simulink model "SF051A_SnsrOffsLrng"  (R2013b)
settings: Solver=FixedStepDiscrete  SolverMode=SingleTasking  StartTime=0.0  StopTime=1  FixedStep=0.002  RelTol=1e-3
undefined symbols (not defined in the file): ARCHGLBPRM_10MILLISEC_SEC_F32, ARCHGLBPRM_2MILLISEC_SEC_F32, ARCHGLBPRM_2PI_ULS_F32, ARCHGLBPRM_FLOATZEROTHD_ULS_F32, ARCHGLBPRM_PIOVER180_ULS_F32, CNV100MICROSECTOMILLISEC_MILLISECPERCNT_F32, CNV100MICROSECTOSEC_SECPERCNT_F32, COVRAMTRXNIT_ULS_F32, HWAUTHYTHD_ULS_F32, HWTQLRNGSTSLRND_CNT_U08, HWTQLRNGSTSNEGOFFS_CNT_U08, HWTQLRNGSTSNOTLRND_CNT_U08, HWTQLRNGSTSPOSOFFS_CNT_U08, HWTQLRNGSTSZEROOFFS_CNT_U08, HWTQLRNGTMRHILIM_SEC_F32, IDYMTRX_ULS_F32, IVS10MS_ULSPERSEC_F32, LRNGFILTICON_ULS_F32, NvmGetErrSts1, ONE_ULS_F32, SnsrOffsLrnd, SnsrOffsLrngFctEna, SnsrOffsLrngHwAgLrngDrvgDstThd, SnsrOffsLrngHwAgLrngEna, SnsrOffsLrngHwAgLrngHwVelThd, SnsrOffsLrngHwAgLrngSysTqThd, SnsrOffsLrngHwAgLrngSysTqThdMed, SnsrOffsLrngHwAgLrngSysTqThdTrustd, SnsrOffsLrngHwAgLrngSysTqThdWide, SnsrOffsLrngHwAgLrngTi, SnsrOffsLrngHwAgLrngVehSpdThd, SnsrOffsLrngHwAgLrngYawOffsDbnd, SnsrOffsLrngHwAgLrngYawRateThd, SnsrOffsLrngHwAgOffsLim, SnsrOffsLrngHwTqLrngEna, SnsrOffsLrngHwTqLrngEnaTiThd, SnsrOffsLrngHwTqLrngHwAgDbnd, SnsrOffsLrngHwTqLrngHwAgThd, SnsrOffsLrngHwTqLrngHwTqThd, SnsrOffsLrngHwTqLrngHwTqZeroOffsThd, SnsrOffsLrngHwTqLrngHwVelThd, SnsrOffsLrngHwTqLrngMeasTi, SnsrOffsLrngHwTqLrngMeasTiScar, SnsrOffsLrngHwTqLrngSampleImbThd1, SnsrOffsLrngHwTqLrngSampleImbThd2, SnsrOffsLrngHwTqLrngSampleThd1, SnsrOffsLrngHwTqLrngSampleThd2, SnsrOffsLrngHwTqLrngTiWghtCoeff, SnsrOffsLrngHwTqLrngVehSpdThd, SnsrOffsLrngHwTqOffsLim, SnsrOffsLrngSampleCntForHwTqLrngRst, SnsrOffsLrngTqInpDetnPwrEstimnThd, SnsrOffsLrngTqInpDetnSinGenrAmp, SnsrOffsLrngTqInpDetnSinGenrFrq, SnsrOffsLrngTqInpDetnStg1FilGain, SnsrOffsLrngTqInpDetnStg1WinSize, SnsrOffsLrngTqInpDetnStg2FilGainCen, SnsrOffsLrngTqInpDetnStg2FilGainDwn, SnsrOffsLrngTqInpDetnStg2FilGainUp, SnsrOffsLrngTqInpDetnStg2WinSize ... (+15)
libraries: Fil x34, FixdToFloat x17, FloatToFixd x16, NxtrLim x15, simulink x12, NxtrAbslt x12, NxtrNvM x8, NxtrMin x5, NxtrMath x3
(part 3 of 11)

== system SF051A_SnsrOffsLrng/SnsrOffsLrng/SetHwAgOffs ==
  note: User wants to force the learned offset to a particular value.  Learning will continue and then
      | be written to NVM at key off as usual.
  HwAgOffs_ArgIn : Inport
  HwAgLrngStRst_ArgIn : Inport  Port=2
  function : TriggerPort  TriggerType=function-call
  Constant1 : Constant  RequirementInfo={'linktype_rmi_doors' '0000babd (/E-STEER Core/SubSystem Specifications/Application Functions/SF051A Sensor Offset Learning)' '#SF051A_230' 'true' 'REQ:SF051A_230' '' } %GIDa_cf4a6147_0323_42ae_80d2_af4f1777b13a  Value=SnsrOffsLrngHwAgOffsLim  OutDataTypeStr=single
  Constant5 : Constant  Value=true  OutDataTypeStr=boolean
      settings: AttributesFormatString=%<OutDataTypeStr>
  Data Store Write : DataStoreWrite  DataStoreName=SnsrOffsLrnd  DataStoreElements=SnsrOffsLrnd.HwAgOffs
  Data Store Write1 : DataStoreWrite  DataStoreName=HwAgLrngStRst
  Do nothing : Subsystem  TreatAsAtomicUnit=on
  FloatToFixd_s16_f32 : FloatToFixd/FloatToFixd_s16_f32  Param1=10
  If : If  IfExpression=u1
  LimDyn_f32 : NxtrLim/LimDyn_f32  RequirementInfo={'linktype_rmi_doors' '0000babd (/E-STEER Core/SubSystem Specifications/Application Functions/SF051A Sensor Offset Learning)' '#SF051A_230' 'true' 'REQ:SF051A_230' '' } %GIDa_5bdd1159_6844_4d61_b5ac_4bd6393bb1d8
  Reset Learning : Subsystem  TreatAsAtomicUnit=on
  Set Ram Block Status : NxtrNvM/Set Ram Block Status  FuncName=Set Ram Block Status  NvMBlockName=SnsrOffsLrnd  VoidFuncRtn=on  BlockChanged_DSN=NvMSRBS_BlockChanged4  Return_DSN=NvMSRBS_Return4
      settings: AttributesFormatString=%<FuncName>
  Subsystem5 : Subsystem  Description=|  mask(Copyright Information){none=on}
      | Copyright info block.                                               
      |                                                                     
      | Place copyright information at the top of every subsystem in design.
      mask prompts: none "No parameters"
      mask help: Place copyright information at the top of every subsystem in design.
      mask Display:
      | NxtrConf = 'Nexteer Confidential';
      | 
      | sys = bdroot; %handle for the current model ("system")
      | first = get_param(sys,'Created');
      | first = first(end-3:end);  %year is last four digits
      | 
      | last = get_param(sys,'LastModifiedDate');
      | if isempty(last)
      |     last = datestr(now,'yyyy');
      | else
      |     last = last(end-3:end);
      | end
      | 
      | if strcmp(first,last)
      |     fprintf('%s -- Copyright %s Nexteer',NxtrConf,first)
      | else
      |     fprintf('%s -- %s%s- %s Nexteer',NxtrConf,char(169),first,last)
      | end
  Unary Minus : UnaryMinus  RequirementInfo={'linktype_rmi_doors' '0000babd (/E-STEER Core/SubSystem Specifications/Application Functions/SF051A Sensor Offset Learning)' '#SF051A_230' 'true' 'REQ:SF051A_230' '' } %GIDa_8391f97f_4728_4542_8e93_eb1d16ca3e52
  wires:
  Constant1/1 -> LimDyn_f32/3, Unary Minus/1
  LimDyn_f32/1 -> [SetHwAgLrngFil1StVari], FloatToFixd_s16_f32/1
  FloatToFixd_s16_f32/1 -> Data Store Write/1
  Constant5/1 -> Set Ram Block Status/1
  Unary Minus/1 -> LimDyn_f32/2
  HwAgOffs_ArgIn/1 -> LimDyn_f32/1
  [SetHwAgLrngFil1StVari] -> Reset Learning/1(SetHwAgLrngFil1StVari)
  If/1 -> Reset Learning/Action
  If/2 -> Do nothing/Action
  HwAgLrngStRst_ArgIn/1 -> Data Store Write1/1, If/1

== system SF051A_SnsrOffsLrng/SnsrOffsLrng/SetHwTqOffs ==
  note: Note for Developer:
      | This version does not have the capability of recovering
      | the last learning state once a "Reset Learning" has been
      | performed.
      | In other words: the Covariance Matriy, the Estimations Vector
      | and the Positive and Negative Counters can no be written
      | using eTool.
  note: User wants to force the learned offset to a particular value.  Learning will continue and then
      | be written to NVM at key off as usual.
  HwTqOffs_ArgIn : Inport
  HwTqLrngStRst_ArgIn : Inport  Port=2
  function : TriggerPort  TriggerType=function-call
  Constant1 : Constant  RequirementInfo={'linktype_rmi_doors' '0000babd (/E-STEER Core/SubSystem Specifications/Application Functions/SF051A Sensor Offset Learning)' '#SF051A_232' 'true' 'REQ:SF051A_232' '' } %GIDa_219fb91a_9c6b_4266_a0e9_012c6c46364f  Value=SnsrOffsLrngHwTqOffsLim  OutDataTypeStr=single
  Constant5 : Constant  Value=true  OutDataTypeStr=boolean
      settings: AttributesFormatString=%<OutDataTypeStr>
  Data Store Write : DataStoreWrite  DataStoreName=SnsrOffsLrnd  DataStoreElements=SnsrOffsLrnd.HwTqOffs
  Data Store Write1 : DataStoreWrite  DataStoreName=HwTqLrngStRst
  Do nothing : Subsystem  TreatAsAtomicUnit=on
  FloatToFixd_s16_f32 : FloatToFixd/FloatToFixd_s16_f32  Param1=12
  If : If  IfExpression=u1
  LimDyn_f32 : NxtrLim/LimDyn_f32  RequirementInfo={'linktype_rmi_doors' '0000babd (/E-STEER Core/SubSystem Specifications/Application Functions/SF051A Sensor Offset Learning)' '#SF051A_232' 'true' 'REQ:SF051A_232' '' } %GIDa_8a55e285_f6d0_4af0_87c3_e1d2354db2fa
  Reset Learning : Subsystem  TreatAsAtomicUnit=on
  Set Ram Block Status : NxtrNvM/Set Ram Block Status  FuncName=Set Ram Block Status  NvMBlockName=SnsrOffsLrnd  VoidFuncRtn=on  BlockChanged_DSN=NvMSRBS_BlockChanged5  Return_DSN=NvMSRBS_Return5
      settings: AttributesFormatString=%<FuncName>
  Subsystem5 : Subsystem  Description=|  mask(Copyright Information){none=on}
      | Copyright info block.                                               
      |                                                                     
      | Place copyright information at the top of every subsystem in design.
      mask prompts: none "No parameters"
      mask help: Place copyright information at the top of every subsystem in design.
      mask Display:
      | NxtrConf = 'Nexteer Confidential';
      | 
      | sys = bdroot; %handle for the current model ("system")
      | first = get_param(sys,'Created');
      | first = first(end-3:end);  %year is last four digits
      | 
      | last = get_param(sys,'LastModifiedDate');
      | if isempty(last)
      |     last = datestr(now,'yyyy');
      | else
      |     last = last(end-3:end);
      | end
      | 
      | if strcmp(first,last)
      |     fprintf('%s -- Copyright %s Nexteer',NxtrConf,first)
      | else
      |     fprintf('%s -- %s%s- %s Nexteer',NxtrConf,char(169),first,last)
      | end
  Unary Minus : UnaryMinus  RequirementInfo={'linktype_rmi_doors' '0000babd (/E-STEER Core/SubSystem Specifications/Application Functions/SF051A Sensor Offset Learning)' '#SF051A_232' 'true' 'REQ:SF051A_232' '' } %GIDa_49082dc0_10d2_4695_96b7_275db381282e
  wires:
  Constant1/1 -> LimDyn_f32/3, Unary Minus/1
  FloatToFixd_s16_f32/1 -> Data Store Write/1
  Constant5/1 -> Set Ram Block Status/1
  Unary Minus/1 -> LimDyn_f32/2
  HwTqOffs_ArgIn/1 -> LimDyn_f32/1
  LimDyn_f32/1 -> FloatToFixd_s16_f32/1
  If/1 -> Reset Learning/Action
  If/2 -> Do nothing/Action
  HwTqLrngStRst_ArgIn/1 -> Data Store Write1/1, If/1

== system SF051A_SnsrOffsLrng/SnsrOffsLrng/SetYawRateOffs ==
  note: User wants to force the learned offset to a particular value.  Learning will continue and then
      | be written to NVM at key off as usual.
  VehYawRateOffs_ArgIn : Inport
  VehYawRateLrngStRst_ArgIn : Inport  Port=2
  function : TriggerPort  TriggerType=function-call
  Constant1 : Constant  RequirementInfo={'linktype_rmi_doors' '0000babd (/E-STEER Core/SubSystem Specifications/Application Functions/SF051A Sensor Offset Learning)' '#SF051A_218' 'true' 'REQ:SF051A_218' '' } %GIDa_ab3e8f4a_b511_4467_8e73_7163cbff4053  Value=SnsrOffsLrngYawRateOffsLim  OutDataTypeStr=single
  Constant5 : Constant  Value=true  OutDataTypeStr=boolean
      settings: AttributesFormatString=%<OutDataTypeStr>
  Data Store Write1 : DataStoreWrite  DataStoreName=VehYawRateLrngStRst
  Do nothing : Subsystem  TreatAsAtomicUnit=on
  FloatToFixd_s16_f32 : FloatToFixd/FloatToFixd_s16_f32  Param1=9
  If : If  IfExpression=u1
  LimDyn_f32 : NxtrLim/LimDyn_f32  RequirementInfo={'linktype_rmi_doors' '0000babd (/E-STEER Core/SubSystem Specifications/Application Functions/SF051A Sensor Offset Learning)' '#SF051A_218' 'true' 'REQ:SF051A_218' '' } %GIDa_7eb17ecc_7acb_4d1e_ab0e_493e23ce8555
  NVM RAM : DataStoreWrite  DataStoreName=SnsrOffsLrnd  DataStoreElements=SnsrOffsLrnd.YawRateOffs
  Reset Learning : Subsystem  TreatAsAtomicUnit=on
  Set Ram Block Status : NxtrNvM/Set Ram Block Status  FuncName=Set Ram Block Status  NvMBlockName=SnsrOffsLrnd  VoidFuncRtn=on  BlockChanged_DSN=NvMSRBS_BlockChanged3  Return_DSN=NvMSRBS_Return3
      settings: AttributesFormatString=%<FuncName>
  Subsystem5 : Subsystem  Description=|  mask(Copyright Information){none=on}
      | Copyright info block.                                               
      |                                                                     
      | Place copyright information at the top of every subsystem in design.
      mask prompts: none "No parameters"
      mask help: Place copyright information at the top of every subsystem in design.
      mask Display:
      | NxtrConf = 'Nexteer Confidential';
      | 
      | sys = bdroot; %handle for the current model ("system")
      | first = get_param(sys,'Created');
      | first = first(end-3:end);  %year is last four digits
      | 
      | last = get_param(sys,'LastModifiedDate');
      | if isempty(last)
      |     last = datestr(now,'yyyy');
      | else
      |     last = last(end-3:end);
      | end
      | 
      | if strcmp(first,last)
      |     fprintf('%s -- Copyright %s Nexteer',NxtrConf,first)
      | else
      |     fprintf('%s -- %s%s- %s Nexteer',NxtrConf,char(169),first,last)
      | end
  Unary Minus : UnaryMinus  RequirementInfo={'linktype_rmi_doors' '0000babd (/E-STEER Core/SubSystem Specifications/Application Functions/SF051A Sensor Offset Learning)' '#SF051A_218' 'true' 'REQ:SF051A_218' '' } %GIDa_9f76f36b_b8a7_4ab3_b85e_9e0995778375
  wires:
  Constant1/1 -> Unary Minus/1, LimDyn_f32/3
  LimDyn_f32/1 -> [SetYawLrngFil1StVari], FloatToFixd_s16_f32/1
  FloatToFixd_s16_f32/1 -> NVM RAM/1
  Constant5/1 -> Set Ram Block Status/1
  Unary Minus/1 -> LimDyn_f32/2
  VehYawRateOffs_ArgIn/1 -> LimDyn_f32/1
  [SetYawLrngFil1StVari] -> Reset Learning/1(SetYawLrngFil1StVari)
  If/1 -> Reset Learning/Action
  If/2 -> Do nothing/Action
  VehYawRateLrngStRst_ArgIn/1 -> Data Store Write1/1, If/1

== system SF051A_SnsrOffsLrng/SnsrOffsLrng/SnsrOffsLrngInit1 ==
  note: Perform KUpdate operations to convert
      | calibrations from Hz to Uls
  note: If NVM is good use it as output.  Otherwise,
      | set stuff to zeros.
  function : TriggerPort  TriggerType=function-call
  Data Store Read : DataStoreRead  DataStoreName=SnsrOffsLrnd  DataStoreElements=SnsrOffsLrnd.HwTqLrngCovariMtrx(:,:)
  Display : Display
  Initialize Filters : Subsystem
  NVM Management : Subsystem
  Subsystem5 : Subsystem  Description=|  mask(Copyright Information){none=on}
      | Copyright info block.                                               
      |                                                                     
      | Place copyright information at the top of every subsystem in design.
      mask prompts: none "No parameters"
      mask help: Place copyright information at the top of every subsystem in design.
      mask Display:
      | NxtrConf = 'Nexteer Confidential';
      | 
      | sys = bdroot; %handle for the current model ("system")
      | first = get_param(sys,'Created');
      | first = first(end-3:end);  %year is last four digits
      | 
      | last = get_param(sys,'LastModifiedDate');
      | if isempty(last)
      |     last = datestr(now,'yyyy');
      | else
      |     last = last(end-3:end);
      | end
      | 
      | if strcmp(first,last)
      |     fprintf('%s -- Copyright %s Nexteer',NxtrConf,first)
      | else
      |     fprintf('%s -- %s%s- %s Nexteer',NxtrConf,char(169),first,last)
      | end
  VehYawRateOffs : Outport
  HwAgOffs : Outport  Port=2
  HwTqOffs : Outport  Port=3
  wires:
  NVM Management/1(VehYawRateOffs) -> VehYawRateOffs/1
  NVM Management/2(HwAgOffs) -> HwAgOffs/1
  NVM Management/3(HwTqOffs) -> HwTqOffs/1
  Data Store Read/1 -> Display/1

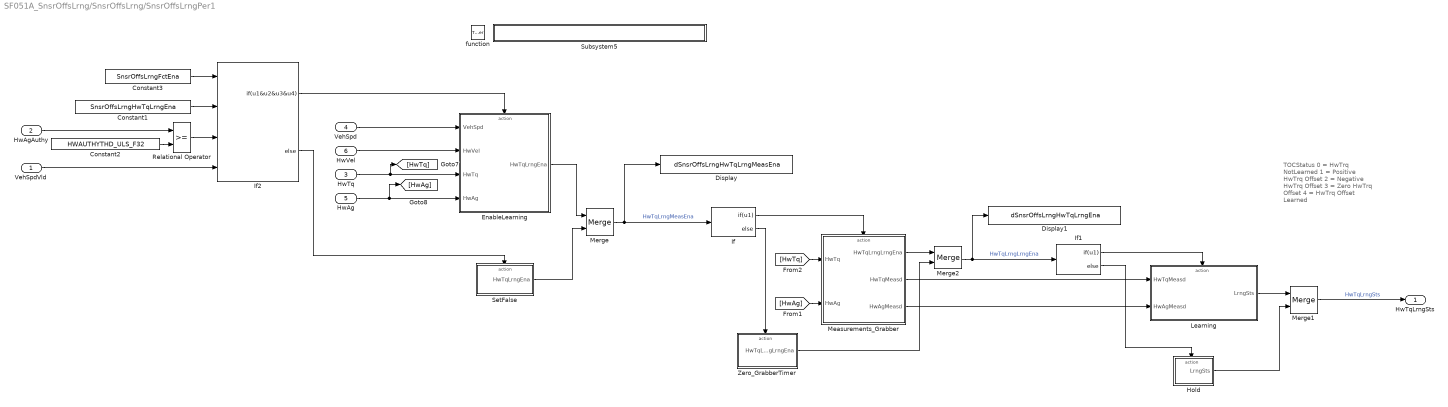
== system SF051A_SnsrOffsLrng/SnsrOffsLrng/SnsrOffsLrngPer1 ==
  note: TOCStatus
      | 0 = HwTrq NotLearned
      | 1 = Positive HwTrq Offset
      | 2 = Negative HwTrq Offset
      | 3 = Zero HwTrq Offset
      | 4 = HwTrq Offset Learned
  VehSpdVld : Inport  RequirementInfo={'linktype_rmi_doors' '0000babd (/E-STEER Core/SubSystem Specifications/Application Functions/SF051A Sensor Offset Learning)' '#SF051A_172' 'true' 'REQ:SF051A_172' '' } %GIDa_4c8f98fb_59b3_4f0f_a449_e0f476a92c6b
  HwAgAuthy : Inport  RequirementInfo={'linktype_rmi_doors' '0000babd (/E-STEER Core/SubSystem Specifications/Application Functions/SF051A Sensor Offset Learning)' '#SF051A_172' 'true' 'REQ:SF051A_172' '' } %GIDa_bc799a18_930e_49aa_970e_d738f90c29be  Port=2
  HwTq : Inport  RequirementInfo={'linktype_rmi_doors' '0000babd (/E-STEER Core/SubSystem Specifications/Application Functions/SF051A Sensor Offset Learning)' '#SF051A_168' 'true' 'REQ:SF051A_168' '' } %GIDa_0cdb420e_6740_4194_bc6e_307440cdb44a  Port=3
  VehSpd : Inport  RequirementInfo={'linktype_rmi_doors' '0000babd (/E-STEER Core/SubSystem Specifications/Application Functions/SF051A Sensor Offset Learning)' '#SF051A_171' 'true' 'REQ:SF051A_171' '' } %GIDa_39046408_4297_4feb_8dd1_f49d24eac858  Port=4
  HwAg : Inport  RequirementInfo={'linktype_rmi_doors' '0000babd (/E-STEER Core/SubSystem Specifications/Application Functions/SF051A Sensor Offset Learning)' '#SF051A_170' 'true' 'REQ:SF051A_170' '' } %GIDa_3e08615c_a8b7_4c69_ae09_e09287af3916  Port=5
  HwVel : Inport  RequirementInfo={'linktype_rmi_doors' '0000babd (/E-STEER Core/SubSystem Specifications/Application Functions/SF051A Sensor Offset Learning)' '#SF051A_169' 'true' 'REQ:SF051A_169' '' } %GIDa_81a5698e_2e55_4c38_b0b0_32579241a4a2  Port=6
  function : TriggerPort  TriggerType=function-call
  Constant1 : Constant  RequirementInfo={'linktype_rmi_doors' '0000babd (/E-STEER Core/SubSystem Specifications/Application Functions/SF051A Sensor Offset Learning)' '#SF051A_149' 'true' 'REQ:SF051A_149' '' ; 'linktype_rmi_doors' '0000babd (/E-STEER Core/SubSystem Specifications/Application Functions/SF051A Sensor Offset Learning)' '#SF051A_172' 'true' 'REQ:SF051A_172' '' } %GIDa_535f024a_9979_46f7_87c9_cdf0e6070b24  Value=SnsrOffsLrngHwTqLrngEna
  Constant2 : Constant  RequirementInfo={'linktype_rmi_doors' '0000babd (/E-STEER Core/SubSystem Specifications/Application Functions/SF051A Sensor Offset Learning)' '#SF051A_172' 'true' 'REQ:SF051A_172' '' } %GIDa_122749e3_4a4e_4ab2_967d_239078c81b67  Value=HWAUTHYTHD_ULS_F32
  Constant3 : Constant  RequirementInfo={'linktype_rmi_doors' '0000babd (/E-STEER Core/SubSystem Specifications/Application Functions/SF051A Sensor Offset Learning)' '#SF051A_26' 'true' 'REQ:SF051A_26' '' } %GIDa_da187dda_b310_4c1b_bb0d_bc714549b8f1  Value=SnsrOffsLrngFctEna
  Display : DataStoreWrite  DataStoreName=dSnsrOffsLrngHwTqLrngMeasEna
  Display1 : DataStoreWrite  DataStoreName=dSnsrOffsLrngHwTqLrngEna
  EnableLearning : Subsystem  RequirementInfo={'linktype_rmi_doors' '0000babd (/E-STEER Core/SubSystem Specifications/Application Functions/SF051A Sensor Offset Learning)' '#SF051A_165' 'true' 'REQ:SF051A_165' '' } %GIDa_b1222e97_8db5_4cd5_9a17_e480f73facda  TreatAsAtomicUnit=on
  Hold : Subsystem  TreatAsAtomicUnit=on
  If : If  RequirementInfo={'linktype_rmi_doors' '0000babd (/E-STEER Core/SubSystem Specifications/Application Functions/SF051A Sensor Offset Learning)' '#SF051A_162' 'true' 'REQ:SF051A_162' '' } %GIDa_ff422a66_a1c6_4a1f_8e22_e07d1158d789  IfExpression=u1
  If1 : If  RequirementInfo={'linktype_rmi_doors' '0000babd (/E-STEER Core/SubSystem Specifications/Application Functions/SF051A Sensor Offset Learning)' '#SF051A_182' 'true' 'REQ:SF051A_182' '' } %GIDa_2b1810eb_40e4_47d2_bf1d_d63a9f5ada2e  IfExpression=u1
  If2 : If  RequirementInfo={'linktype_rmi_doors' '0000babd (/E-STEER Core/SubSystem Specifications/Application Functions/SF051A Sensor Offset Learning)' '#SF051A_172' 'true' 'REQ:SF051A_172' '' ; 'linktype_rmi_doors' '0000babd (/E-STEER Core/SubSystem Specifications/Application Functions/SF051A Sensor Offset Learning)' '#SF051A_26' 'true' 'REQ:SF051A_26' '' } %GIDa_c02bc2c0_3e44_40e5_864a_39991bb27631  NumInputs=4  IfExpression=u1&u2&u3&u4
  Learning : Subsystem  RequirementInfo={'linktype_rmi_doors' '0000babd (/E-STEER Core/SubSystem Specifications/Application Functions/SF051A Sensor Offset Learning)' '#SF051A_167' 'true' 'REQ:SF051A_167' '' ; 'linktype_rmi_doors' '0000babd (/E-STEER Core/SubSystem Specifications/Application Functions/SF051A Sensor Offset Learning)' '#SF051A_152' 'true' 'REQ:SF051A_152' '' } %GIDa_1b59b871_a124_470c_ac32_3b22f2dc3167  TreatAsAtomicUnit=on
  Measurements_Grabber : Subsystem  RequirementInfo={'linktype_rmi_doors' '0000babd (/E-STEER Core/SubSystem Specifications/Application Functions/SF051A Sensor Offset Learning)' '#SF051A_163' 'true' 'REQ:SF051A_163' '' } %GIDa_6482af8e_2bfa_4ab1_8618_42b9ef0606fb  TreatAsAtomicUnit=on
  Merge : Merge
  Merge1 : Merge
  Merge2 : Merge
  Relational Operator : RelationalOperator  RequirementInfo={'linktype_rmi_doors' '0000babd (/E-STEER Core/SubSystem Specifications/Application Functions/SF051A Sensor Offset Learning)' '#SF051A_172' 'true' 'REQ:SF051A_172' '' } %GIDa_037935c3_3c71_42e9_a97d_8c93dc2f08bc  OutDataTypeStr=boolean
  SetFalse : Subsystem  TreatAsAtomicUnit=on
  Subsystem5 : Subsystem  Description=|  mask(Copyright Information){none=on}
      | Copyright info block.                                               
      |                                                                     
      | Place copyright information at the top of every subsystem in design.
      mask prompts: none "No parameters"
      mask help: Place copyright information at the top of every subsystem in design.
      mask Display:
      | NxtrConf = 'Nexteer Confidential';
      | 
      | sys = bdroot; %handle for the current model ("system")
      | first = get_param(sys,'Created');
      | first = first(end-3:end);  %year is last four digits
      | 
      | last = get_param(sys,'LastModifiedDate');
      | if isempty(last)
      |     last = datestr(now,'yyyy');
      | else
      |     last = last(end-3:end);
      | end
      | 
      | if strcmp(first,last)
      |     fprintf('%s -- Copyright %s Nexteer',NxtrConf,first)
      | else
      |     fprintf('%s -- %s%s- %s Nexteer',NxtrConf,char(169),first,last)
      | end
  Zero_GrabberTimer : Subsystem  TreatAsAtomicUnit=on
  HwTqLrngSts : Outport
  wires:
  Relational Operator/1 -> If2/3
  VehSpdVld/1 -> If2/4
  HwAgAuthy/1 -> Relational Operator/1
  Constant2/1 -> Relational Operator/2
  Constant3/1 -> If2/1
  VehSpd/1 -> EnableLearning/1(VehSpd)
  HwVel/1 -> EnableLearning/2(HwVel)
  If/1 -> Measurements_Grabber/Action
  If/2 -> Zero_GrabberTimer/Action
  Measurements_Grabber/1(HwTqLrngLrngEna) -> Merge2/1
  Measurements_Grabber/2(" HwTqMeasd") -> Learning/1(HwTqMeasd)
  Measurements_Grabber/3(HwAgMeasd) -> Learning/2(HwAgMeasd)
  If1/1 -> Learning/Action
  Merge1/1 -> HwTqLrngSts/1  "HwTqLrngSts"
  Constant1/1 -> If2/2
  If2/1 -> EnableLearning/Action
  If2/2 -> SetFalse/Action
  SetFalse/1(HwTqLrngEna) -> Merge/2
  EnableLearning/1(HwTqLrngEna) -> Merge/1
  Merge/1 -> If/1, Display/1  "HwTqLrngMeasEna"
  If1/2 -> Hold/Action
  Learning/1(LrngSts) -> Merge1/1
  Hold/1(LrngSts) -> Merge1/2
  [HwAg] -> Measurements_Grabber/2(HwAg)
  [HwTq] -> Measurements_Grabber/1(HwTq)
  Merge2/1 -> Display1/1, If1/1  "HwTqLrngLrngEna"
  Zero_GrabberTimer/1(HwTqLrngLrngEna) -> Merge2/2
  HwTq/1 -> [HwTq], EnableLearning/3(HwTq)
  HwAg/1 -> [HwAg], EnableLearning/4(HwAg)

== system SF051A_SnsrOffsLrng/SnsrOffsLrng/SnsrOffsLrngPer2 ==
  VehSpd : Inport
  HwAg : Inport  Port=2
  VehYawRate : Inport  Port=3
  HwVel : Inport  Port=4
  HwTq : Inport  Port=5
  MotTqCmdCrf : Inport  Port=6
  VehYawRateVld : Inport  Port=7
  HwAgAuthy : Inport  Port=8
  VehSpedVld : Inport  Port=9
  HwTqLrngSts : Inport  Port=10
  function : TriggerPort  TriggerType=function-call
  Constant : Constant  RequirementInfo={'linktype_rmi_doors' '0000babd (/E-STEER Core/SubSystem Specifications/Application Functions/SF051A Sensor Offset Learning)' '#SF051A_26' 'true' 'REQ:SF051A_26' '' } %GIDa_87a2c3d1_22c0_4f41_9628_e13acbd87715  Value=SnsrOffsLrngFctEna
  Do nothing : Subsystem  TreatAsAtomicUnit=on
  Enable_Function : Subsystem  TreatAsAtomicUnit=on
  If : If  RequirementInfo={'linktype_rmi_doors' '0000babd (/E-STEER Core/SubSystem Specifications/Application Functions/SF051A Sensor Offset Learning)' '#SF051A_26' 'true' 'REQ:SF051A_26' '' } %GIDa_ccb961ec_3e2e_4777_9fe3_5289931ee51d  IfExpression=u1
  Subsystem5 : Subsystem  Description=|  mask(Copyright Information){none=on}
      | Copyright info block.                                               
      |                                                                     
      | Place copyright information at the top of every subsystem in design.
      mask prompts: none "No parameters"
      mask help: Place copyright information at the top of every subsystem in design.
      mask Display:
      | NxtrConf = 'Nexteer Confidential';
      | 
      | sys = bdroot; %handle for the current model ("system")
      | first = get_param(sys,'Created');
      | first = first(end-3:end);  %year is last four digits
      | 
      | last = get_param(sys,'LastModifiedDate');
      | if isempty(last)
      |     last = datestr(now,'yyyy');
      | else
      |     last = last(end-3:end);
      | end
      | 
      | if strcmp(first,last)
      |     fprintf('%s -- Copyright %s Nexteer',NxtrConf,first)
      | else
      |     fprintf('%s -- %s%s- %s Nexteer',NxtrConf,char(169),first,last)
      | end
  wires:
  VehSpd/1 -> Enable_Function/1(VehSpd)
  HwAg/1 -> Enable_Function/2(HwAg)
  VehYawRate/1 -> Enable_Function/3(VehYawRate)
  HwVel/1 -> Enable_Function/4(HwVel)
  HwTq/1 -> Enable_Function/5(HwTq)
  MotTqCmdCrf/1 -> Enable_Function/6(MotTqCmdCrf)
  VehYawRateVld/1 -> Enable_Function/7(VehYawRateVld)
  HwAgAuthy/1 -> Enable_Function/8(HwAgAuthy)
  VehSpedVld/1 -> Enable_Function/9(VehSpedVld)
  HwTqLrngSts/1 -> Enable_Function/10(HwTqLrngSts)
  Constant/1 -> If/1
  If/1 -> Enable_Function/Action
  If/2 -> Do nothing/Action

== system SF051A_SnsrOffsLrng/SnsrOffsLrng/Subsystem5 ==

== system SF051A_SnsrOffsLrng/call_SnsrOffsLrngInit1/Subsystem5 ==

== system SF051A_SnsrOffsLrng/call_SnsrOffsLrngPer1/Subsystem5 ==

== system SF051A_SnsrOffsLrng/call_SnsrOffsLrngPer2/Subsystem5 ==

== system SF051A_SnsrOffsLrng/SnsrOffsLrng/GetHwAgOffs/Subsystem5 ==

== system SF051A_SnsrOffsLrng/SnsrOffsLrng/GetHwTqOffs/Subsystem5 ==

== system SF051A_SnsrOffsLrng/SnsrOffsLrng/GetYawRateOffs/Subsystem5 ==

== system SF051A_SnsrOffsLrng/SnsrOffsLrng/RstHwTq/GetRefTmr100MicroSec32bit ==
  note: 1 count = 100 uSec
  note: seconds
  note: microseconds
  note: counts
  note: Wrap-to-zero
  note: GetRefTmr100MicroSec32bit
  note: Created Aug 18, 2015
      | Modified Oct 21, 2015
      | Modified Oct 30, 2015
      | Kevin Derry
  CopyRight2 : Subsystem  Description=|  mask(Copyright Information){none=on}
      | Copyright info block.                                               
      |                                                                     
      | Place copyright information at the top of every subsystem in design.
      mask prompts: none "No parameters"
      mask help: Place copyright information at the top of every subsystem in design.
      mask Display:
      | NxtrConf = 'Nexteer Confidential';
      | 
      | sys = bdroot; %handle for the current model ("system")
      | first = get_param(sys,'Created');
      | if(isempty(first))
      |     first = datestr(now,'yyyy');
      | else
      |     first = first(end-3:end);  %year is last four digits
      | end
      | 
      | last = get_param(sys,'LastModifiedDate');
      | if isempty(last)
      |     last = datestr(now,'yyyy');
      | else
      |     last = last(end-3:end);
      | end
      | 
      | if strcmp(first,last)
      |     fprintf('%s -- Copyright %s Nexteer',NxtrConf,first)
      | else
      |     fprintf('%s -- %s%s- %s Nexteer',NxtrConf,char(169),first,last)
      | end
  Count per uSec : Constant  Value=0.01
  Data Store Read1 : DataStoreRead  DataStoreName=SimnTi
  Data Type Conversion1 : DataTypeConversion  OutDataTypeStr=uint32
  Divide1 : Product  Inputs=**
  Divide2 : Product  Inputs=*/
  Max Counts : Constant  Value=2^32-1
  Product1 : Product
  Product2 : Product
  Rounding : Rounding
  Subtract1 : Sum  Inputs=+-
  uSec per Sec : Constant  Value=1000000
  RefTmr : Outport
  wires:
  Product2/1 -> Subtract1/2
  Subtract1/1 -> Data Type Conversion1/1
  Rounding/1 -> Product2/1
  Divide2/1 -> Rounding/1
  Max Counts/1 -> Divide2/2, Product2/2
  Divide1/1 -> Divide2/1, Subtract1/1
  Product1/1 -> Divide1/1
  Count per uSec/1 -> Divide1/2
  uSec per Sec/1 -> Product1/2
  Data Type Conversion1/1 -> RefTmr/1
  Data Store Read1/1 -> Product1/1

== system SF051A_SnsrOffsLrng/SnsrOffsLrng/RstHwTq/Subsystem5 ==

== system SF051A_SnsrOffsLrng/SnsrOffsLrng/RstYawAndAg/Subsystem5 ==

== system SF051A_SnsrOffsLrng/SnsrOffsLrng/SetHwAgOffs/Do nothing ==
  Action Port : ActionPort  ActionType=else
  Subsystem5 : Subsystem  Description=|  mask(Copyright Information){none=on}
      | Copyright info block.                                               
      |                                                                     
      | Place copyright information at the top of every subsystem in design.
      mask prompts: none "No parameters"
      mask help: Place copyright information at the top of every subsystem in design.
      mask Display:
      | NxtrConf = 'Nexteer Confidential';
      | 
      | sys = bdroot; %handle for the current model ("system")
      | first = get_param(sys,'Created');
      | first = first(end-3:end);  %year is last four digits
      | 
      | last = get_param(sys,'LastModifiedDate');
      | if isempty(last)
      |     last = datestr(now,'yyyy');
      | else
      |     last = last(end-3:end);
      | end
      | 
      | if strcmp(first,last)
      |     fprintf('%s -- Copyright %s Nexteer',NxtrConf,first)
      | else
      |     fprintf('%s -- %s%s- %s Nexteer',NxtrConf,char(169),first,last)
      | end

== system SF051A_SnsrOffsLrng/SnsrOffsLrng/SetHwAgOffs/Reset Learning ==
  SetHwAgLrngFil1StVari : Inport
  Action Port : ActionPort  ActionType=then
  Constant : Constant  Value=ZERO_ULS_F32  OutDataTypeStr=single
      settings: AttributesFormatString=%<OutDataTypeStr>
  Constant1 : Constant  Value=ZERO_ULS_F32  OutDataTypeStr=single
      settings: AttributesFormatString=%<OutDataTypeStr>
  Constant2 : Constant  Value=0  OutDataTypeStr=int16
      settings: AttributesFormatString=%<OutDataTypeStr>
  Data Store Write : DataStoreWrite  DataStoreName=HwAgLrngFil1  DataStoreElements=HwAgLrngFil1.FilSt
  Data Store Write1 : DataStoreWrite  DataStoreName=HwAgLrngSysTqFil1  DataStoreElements=HwAgLrngSysTqFil1.FilSt
  Data Store Write2 : DataStoreWrite  DataStoreName=SnsrOffsLrnd  DataStoreElements=SnsrOffsLrnd.HwAgLrndTi#SnsrOffsLrnd.HwAgLrngHwAgFilSt#SnsrOffsLrnd.HwAgLrngSysTqFilSt#SnsrOffsLrnd.HwAgLrngYawOffsRef
  Data Store Write3 : DataStoreWrite  DataStoreName=HwAgLrngFil2  DataStoreElements=HwAgLrngFil2.FilSt
  Data Store Write4 : DataStoreWrite  DataStoreName=HwAgLrngSysTqFil2  DataStoreElements=HwAgLrngSysTqFil2.FilSt
  NVM Read : DataStoreRead  DataStoreName=SnsrOffsLrnd  DataStoreElements=SnsrOffsLrnd.YawRateOffs
  Subsystem5 : Subsystem  Description=|  mask(Copyright Information){none=on}
      | Copyright info block.                                               
      |                                                                     
      | Place copyright information at the top of every subsystem in design.
      mask prompts: none "No parameters"
      mask help: Place copyright information at the top of every subsystem in design.
      mask Display:
      | NxtrConf = 'Nexteer Confidential';
      | 
      | sys = bdroot; %handle for the current model ("system")
      | first = get_param(sys,'Created');
      | first = first(end-3:end);  %year is last four digits
      | 
      | last = get_param(sys,'LastModifiedDate');
      | if isempty(last)
      |     last = datestr(now,'yyyy');
      | else
      |     last = last(end-3:end);
      | end
      | 
      | if strcmp(first,last)
      |     fprintf('%s -- Copyright %s Nexteer',NxtrConf,first)
      | else
      |     fprintf('%s -- %s%s- %s Nexteer',NxtrConf,char(169),first,last)
      | end
  wires:
  SetHwAgLrngFil1StVari/1 -> Data Store Write3/1, Data Store Write/1
  Constant/1 -> Data Store Write4/1, Data Store Write1/1
  Constant1/1 -> Data Store Write2/1
  NVM Read/1 -> Data Store Write2/4
  Constant2/1 -> Data Store Write2/3, Data Store Write2/2

== system SF051A_SnsrOffsLrng/SnsrOffsLrng/SetHwAgOffs/Subsystem5 ==

== system SF051A_SnsrOffsLrng/SnsrOffsLrng/SetHwTqOffs/Do nothing ==
  Action Port : ActionPort  ActionType=else
  Subsystem5 : Subsystem  Description=|  mask(Copyright Information){none=on}
      | Copyright info block.                                               
      |                                                                     
      | Place copyright information at the top of every subsystem in design.
      mask prompts: none "No parameters"
      mask help: Place copyright information at the top of every subsystem in design.
      mask Display:
      | NxtrConf = 'Nexteer Confidential';
      | 
      | sys = bdroot; %handle for the current model ("system")
      | first = get_param(sys,'Created');
      | first = first(end-3:end);  %year is last four digits
      | 
      | last = get_param(sys,'LastModifiedDate');
      | if isempty(last)
      |     last = datestr(now,'yyyy');
      | else
      |     last = last(end-3:end);
      | end
      | 
      | if strcmp(first,last)
      |     fprintf('%s -- Copyright %s Nexteer',NxtrConf,first)
      | else
      |     fprintf('%s -- %s%s- %s Nexteer',NxtrConf,char(169),first,last)
      | end

== system SF051A_SnsrOffsLrng/SnsrOffsLrng/SetHwTqOffs/Reset Learning ==
  note: LPFs
  note: State Variables
  note: NVM
  Action Port : ActionPort  ActionType=then
  Constant1 : Constant  Value=ZERO_ULS_F32  OutDataTypeStr=single
      settings: AttributesFormatString=%<OutDataTypeStr>
  Constant10 : Constant  Value=true  OutDataTypeStr=boolean
      settings: AttributesFormatString=%<OutDataTypeStr>
  Constant3 : Constant  Value=SYSGLBPRM_HWAGHILIM_HWDEG_F32  OutDataTypeStr=single
      settings: AttributesFormatString=%<OutDataTypeStr>
  Constant4 : Constant  Value=IDYMTRX_ULS_F32  VectorParams1D=off  OutDataTypeStr=single
      settings: AttributesFormatString=%<OutDataTypeStr>, 3x3
  Constant5 : Constant  Value=0  OutDataTypeStr=uint16
      settings: AttributesFormatString=%<OutDataTypeStr>
  Constant6 : Constant  Value=0  OutDataTypeStr=uint8
      settings: AttributesFormatString=%<OutDataTypeStr>
  Constant7 : Constant  Value=ZEROVECT_ULS_F32  VectorParams1D=off  OutDataTypeStr=single
      settings: AttributesFormatString=%<OutDataTypeStr>, 3x1
  Constant8 : Constant  Value=COVRAMTRXNIT_ULS_F32  OutDataTypeStr=single
      settings: AttributesFormatString=%<OutDataTypeStr>
  Constant9 : Constant  Value=false  OutDataTypeStr=boolean
      settings: AttributesFormatString=%<OutDataTypeStr>
  Data Store Write1 : DataStoreWrite  DataStoreName=HwTqLrngEnaTmrRef
  Data Store Write10 : DataStoreWrite  DataStoreName=HwTqLrngTqInpPrsnt
  Data Store Write2 : DataStoreWrite  DataStoreName=HwTqLrngMeasTmrRef
  Data Store Write4 : DataStoreWrite  DataStoreName=HwAgMeasFil1  DataStoreElements=HwAgMeasFil1.FilSt
  Data Store Write5 : DataStoreWrite  DataStoreName=HwAgMeasFil2  DataStoreElements=HwAgMeasFil2.FilSt
  Data Store Write6 : DataStoreWrite  DataStoreName=HwTqMeasFil1  DataStoreElements=HwTqMeasFil1.FilSt
  Data Store Write7 : DataStoreWrite  DataStoreName=HwTqMeasFil2  DataStoreElements=HwTqMeasFil2.FilSt
  Data Store Write8 : DataStoreWrite  DataStoreName=HwTqLrngTqInpDetnEnaPrev
  Data Store Write9 : DataStoreWrite  DataStoreName=TqInpDetnHwTqFil  DataStoreElements=TqInpDetnHwTqFil.FilSt
  FloatToFixd_s16_f32 : FloatToFixd/FloatToFixd_s16_f32  Param1=4
  GetRefTmr100MicroSec32bit : Subsystem
  Product : Product
  Subsystem5 : Subsystem  Description=|  mask(Copyright Information){none=on}
      | Copyright info block.                                               
      |                                                                     
      | Place copyright information at the top of every subsystem in design.
      mask prompts: none "No parameters"
      mask help: Place copyright information at the top of every subsystem in design.
      mask Display:
      | NxtrConf = 'Nexteer Confidential';
      | 
      | sys = bdroot; %handle for the current model ("system")
      | first = get_param(sys,'Created');
      | first = first(end-3:end);  %year is last four digits
      | 
      | last = get_param(sys,'LastModifiedDate');
      | if isempty(last)
      |     last = datestr(now,'yyyy');
      | else
      |     last = last(end-3:end);
      | end
      | 
      | if strcmp(first,last)
      |     fprintf('%s -- Copyright %s Nexteer',NxtrConf,first)
      | else
      |     fprintf('%s -- %s%s- %s Nexteer',NxtrConf,char(169),first,last)
      | end
  Update NVM RAM : DataStoreWrite  DataStoreName=SnsrOffsLrnd  DataStoreElements=SnsrOffsLrnd.HwTqLrngSampleCntNeg#SnsrOffsLrnd.HwTqLrngSampleCntPos#SnsrOffsLrnd.HwTqLrngSts#SnsrOffsLrnd.HwTqLrngHwAgRef#SnsrOffsLrnd.HwTqLrngEstimnVect(:,:)#SnsrOffsLrnd.HwTqLrngCovariMtrx(:,:)
  wires:
  Constant1/1 -> Data Store Write9/1, Data Store Write7/1, Data Store Write6/1, Data Store Write5/1, Data Store Write4/1
  GetRefTmr100MicroSec32bit/1(RefTmr) -> Data Store Write2/1, Data Store Write1/1
  Constant3/1 -> FloatToFixd_s16_f32/1
  Constant5/1 -> Update NVM RAM/2, Update NVM RAM/1
  Constant6/1 -> Update NVM RAM/3
  Constant7/1 -> Update NVM RAM/5
  Constant4/1 -> Product/1
  Constant8/1 -> Product/2
  Product/1 -> Update NVM RAM/6
  Constant9/1 -> Data Store Write8/1
  Constant10/1 -> Data Store Write10/1
  FloatToFixd_s16_f32/1 -> Update NVM RAM/4

== system SF051A_SnsrOffsLrng/SnsrOffsLrng/SetHwTqOffs/Subsystem5 ==

== system SF051A_SnsrOffsLrng/SnsrOffsLrng/SetYawRateOffs/Do nothing ==
  Action Port : ActionPort  ActionType=else
  Subsystem5 : Subsystem  Description=|  mask(Copyright Information){none=on}
      | Copyright info block.                                               
      |                                                                     
      | Place copyright information at the top of every subsystem in design.
      mask prompts: none "No parameters"
      mask help: Place copyright information at the top of every subsystem in design.
      mask Display:
      | NxtrConf = 'Nexteer Confidential';
      | 
      | sys = bdroot; %handle for the current model ("system")
      | first = get_param(sys,'Created');
      | first = first(end-3:end);  %year is last four digits
      | 
      | last = get_param(sys,'LastModifiedDate');
      | if isempty(last)
      |     last = datestr(now,'yyyy');
      | else
      |     last = last(end-3:end);
      | end
      | 
      | if strcmp(first,last)
      |     fprintf('%s -- Copyright %s Nexteer',NxtrConf,first)
      | else
      |     fprintf('%s -- %s%s- %s Nexteer',NxtrConf,char(169),first,last)
      | end

== system SF051A_SnsrOffsLrng/SnsrOffsLrng/SetYawRateOffs/Reset Learning ==
  note: Length of time since last learned.
  note: Length of time spent learning.
  SetYawLrngFil1StVari : Inport
  Action Port : ActionPort  ActionType=then
  Constant : Constant  Value=ZERO_ULS_F32  OutDataTypeStr=single
      settings: AttributesFormatString=%<OutDataTypeStr>
  Data Store Write1 : DataStoreWrite  DataStoreName=YawLrngElpdLrngTi
  Data Store Write2 : DataStoreWrite  DataStoreName=SnsrOffsLrnd  DataStoreElements=SnsrOffsLrnd.YawRateElpdTi
  Data Store Write3 : DataStoreWrite  DataStoreName=YawLrngFil2  DataStoreElements=YawLrngFil2.FilSt
  Data Store Write4 : DataStoreWrite  DataStoreName=YawLrngFil1  DataStoreElements=YawLrngFil1.FilSt
  Subsystem5 : Subsystem  Description=|  mask(Copyright Information){none=on}
      | Copyright info block.                                               
      |                                                                     
      | Place copyright information at the top of every subsystem in design.
      mask prompts: none "No parameters"
      mask help: Place copyright information at the top of every subsystem in design.
      mask Display:
      | NxtrConf = 'Nexteer Confidential';
      | 
      | sys = bdroot; %handle for the current model ("system")
      | first = get_param(sys,'Created');
      | first = first(end-3:end);  %year is last four digits
      | 
      | last = get_param(sys,'LastModifiedDate');
      | if isempty(last)
      |     last = datestr(now,'yyyy');
      | else
      |     last = last(end-3:end);
      | end
      | 
      | if strcmp(first,last)
      |     fprintf('%s -- Copyright %s Nexteer',NxtrConf,first)
      | else
      |     fprintf('%s -- %s%s- %s Nexteer',NxtrConf,char(169),first,last)
      | end
  wires:
  SetYawLrngFil1StVari/1 -> Data Store Write3/1, Data Store Write4/1
  Constant/1 -> Data Store Write2/1, Data Store Write1/1

== system SF051A_SnsrOffsLrng/SnsrOffsLrng/SetYawRateOffs/Subsystem5 ==

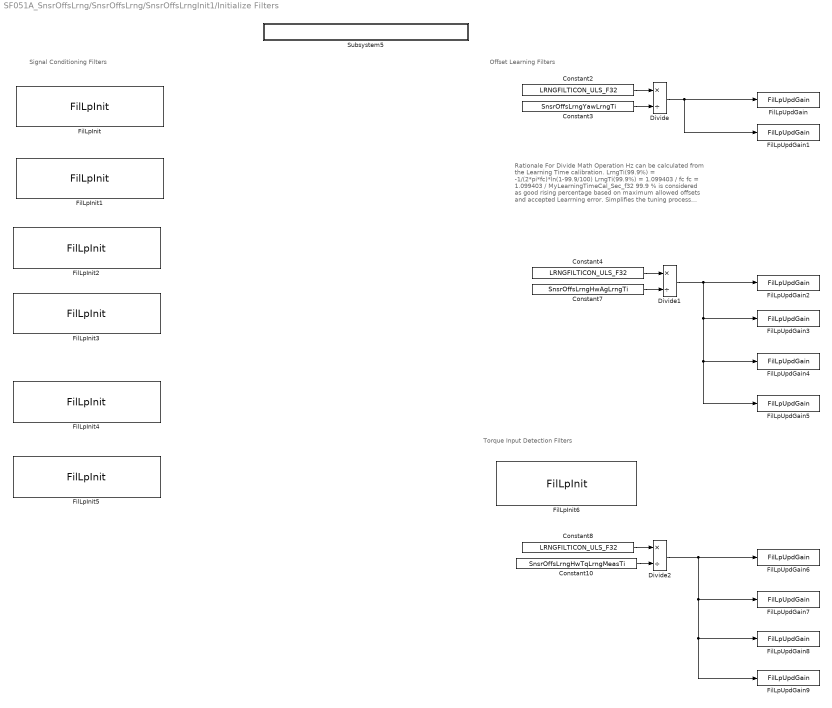
== system SF051A_SnsrOffsLrng/SnsrOffsLrng/SnsrOffsLrngInit1/Initialize Filters ==
  note: Rationale For Divide Math Operation
      |   Hz can be calculated from the Learning Time calibration.
      |   LrngTi(99.9%) = -1/(2*pi*fc)*ln(1-99.9/100)
      |   LrngTi(99.9%) = 1.099403 / fc
      |   fc = 1.099403 / MyLearningTimeCal_Sec_f32
      |
      |   99.9 % is considered as good rising percentage based on
      |   maximum allowed offsets and accepted Learrning error.
      |   Simplifies the tuning process and prevents the customer to
      |   directly find out that we use LPF as the learning method.
  note: Signal Conditioning Filters
  note: Offset Learning Filters
  note: Torque Input Detection Filters
  Constant10 : Constant  Value=SnsrOffsLrngHwTqLrngMeasTi
  Constant2 : Constant  Value=LRNGFILTICON_ULS_F32
  Constant3 : Constant  Value=SnsrOffsLrngYawLrngTi
  Constant4 : Constant  Value=LRNGFILTICON_ULS_F32
  Constant7 : Constant  Value=SnsrOffsLrngHwAgLrngTi
  Constant8 : Constant  Value=LRNGFILTICON_ULS_F32
  Divide : Product  Inputs=*/
  Divide1 : Product  Inputs=*/
  Divide2 : Product  Inputs=*/
  FilLpInit : Fil/FilLpInit  Ic=0  Ts=ARCHGLBPRM_10MILLISEC_SEC_F32  Freq=SnsrOffsLrngYawRateCdngFilFrq  StVar=YawCdngFil1
  FilLpInit1 : Fil/FilLpInit  Ic=0  Ts=ARCHGLBPRM_10MILLISEC_SEC_F32  Freq=SnsrOffsLrngYawRateCdngFilFrq  StVar=YawCdngFil2
  FilLpInit2 : Fil/FilLpInit  Ic=0  Ts=ARCHGLBPRM_10MILLISEC_SEC_F32  Freq=SnsrOffsLrngYawACdngFilFrq  StVar=YawACdngFil
  FilLpInit3 : Fil/FilLpInit  Ic=0  Ts=ARCHGLBPRM_10MILLISEC_SEC_F32  Freq=SnsrOffsLrngTqAndAgFilFrq  StVar=HwAgCdngFil
  FilLpInit4 : Fil/FilLpInit  Ic=0  Ts=ARCHGLBPRM_10MILLISEC_SEC_F32  Freq=SnsrOffsLrngHwVelFilFrq  StVar=HwVelCdngFil
  FilLpInit5 : Fil/FilLpInit  Ic=0  Ts=ARCHGLBPRM_10MILLISEC_SEC_F32  Freq=SnsrOffsLrngTqAndAgFilFrq  StVar=SysTqCdngFil
  FilLpInit6 : Fil/FilLpInit  Ic=0  Ts=ARCHGLBPRM_2MILLISEC_SEC_F32  Freq=SnsrOffsLrngTqInpDetnHwTqFilFrq  StVar=TqInpDetnHwTqFil
  FilLpUpdGain : Fil/FilLpUpdGain  Ts=ARCHGLBPRM_10MILLISEC_SEC_F32  StVar=YawLrngFil1
      settings: AttributesFormatString=|
      | Ts: %<Ts>
      | StVar: %<StVar>
  FilLpUpdGain1 : Fil/FilLpUpdGain  Ts=ARCHGLBPRM_10MILLISEC_SEC_F32  StVar=YawLrngFil2
      settings: AttributesFormatString=|
      | Ts: %<Ts>
      | StVar: %<StVar>
  FilLpUpdGain2 : Fil/FilLpUpdGain  Ts=ARCHGLBPRM_10MILLISEC_SEC_F32  StVar=HwAgLrngFil1
      settings: AttributesFormatString=|
      | Ts: %<Ts>
      | StVar: %<StVar>
  FilLpUpdGain3 : Fil/FilLpUpdGain  Ts=ARCHGLBPRM_10MILLISEC_SEC_F32  StVar=HwAgLrngFil2
      settings: AttributesFormatString=|
      | Ts: %<Ts>
      | StVar: %<StVar>
  FilLpUpdGain4 : Fil/FilLpUpdGain  Ts=ARCHGLBPRM_10MILLISEC_SEC_F32  StVar=HwAgLrngSysTqFil1
      settings: AttributesFormatString=|
      | Ts: %<Ts>
      | StVar: %<StVar>
  FilLpUpdGain5 : Fil/FilLpUpdGain  Ts=ARCHGLBPRM_10MILLISEC_SEC_F32  StVar=HwAgLrngSysTqFil2
      settings: AttributesFormatString=|
      | Ts: %<Ts>
      | StVar: %<StVar>
  FilLpUpdGain6 : Fil/FilLpUpdGain  Ts=ARCHGLBPRM_2MILLISEC_SEC_F32  StVar=HwTqMeasFil1
      settings: AttributesFormatString=|
      | Ts: %<Ts>
      | StVar: %<StVar>
  FilLpUpdGain7 : Fil/FilLpUpdGain  Ts=ARCHGLBPRM_2MILLISEC_SEC_F32  StVar=HwTqMeasFil2
      settings: AttributesFormatString=|
      | Ts: %<Ts>
      | StVar: %<StVar>
  FilLpUpdGain8 : Fil/FilLpUpdGain  Ts=ARCHGLBPRM_2MILLISEC_SEC_F32  StVar=HwAgMeasFil1
      settings: AttributesFormatString=|
      | Ts: %<Ts>
      | StVar: %<StVar>
  FilLpUpdGain9 : Fil/FilLpUpdGain  Ts=ARCHGLBPRM_2MILLISEC_SEC_F32  StVar=HwAgMeasFil2
      settings: AttributesFormatString=|
      | Ts: %<Ts>
      | StVar: %<StVar>
  Subsystem5 : Subsystem  Description=|  mask(Copyright Information){none=on}
      | Copyright info block.                                               
      |                                                                     
      | Place copyright information at the top of every subsystem in design.
      mask prompts: none "No parameters"
      mask help: Place copyright information at the top of every subsystem in design.
      mask Display:
      | NxtrConf = 'Nexteer Confidential';
      | 
      | sys = bdroot; %handle for the current model ("system")
      | first = get_param(sys,'Created');
      | first = first(end-3:end);  %year is last four digits
      | 
      | last = get_param(sys,'LastModifiedDate');
      | if isempty(last)
      |     last = datestr(now,'yyyy');
      | else
      |     last = last(end-3:end);
      | end
      | 
      | if strcmp(first,last)
      |     fprintf('%s -- Copyright %s Nexteer',NxtrConf,first)
      | else
      |     fprintf('%s -- %s%s- %s Nexteer',NxtrConf,char(169),first,last)
      | end
  wires:
  Constant2/1 -> Divide/1
  Constant3/1 -> Divide/2
  Constant4/1 -> Divide1/1
  Constant7/1 -> Divide1/2
  Divide/1 -> FilLpUpdGain1/1, FilLpUpdGain/1
  Constant8/1 -> Divide2/1
  Constant10/1 -> Divide2/2
  Divide2/1 -> FilLpUpdGain9/1, FilLpUpdGain8/1, FilLpUpdGain7/1, FilLpUpdGain6/1
  Divide1/1 -> FilLpUpdGain5/1, FilLpUpdGain4/1, FilLpUpdGain3/1, FilLpUpdGain2/1
